simulink model "BLDC_Final"  (R2021b)
settings: Solver=odeN  StartTime=0.0  StopTime=5  MaxStep=Ts_motor  RelTol=1e-3  EnableMultiTasking=on
InitFcn:
  | load bldcData
model workspace (MAT data in the model file):
  encoderResolution = 2000
  hallOffset = '0.5'
  indexOffset = 850
  polePairs = '4'
undefined symbols (not defined in the file): DiscIntNeverNeededParam, Ts_motor, X, Y, Z
libraries: nesl_utility x23, ee_lib x8, fl_lib x8, sm_lib x7, spsPWMGeneratorDCDCLib x1, slpidlib x1, simulink_extras x1
(part 2 of 2)

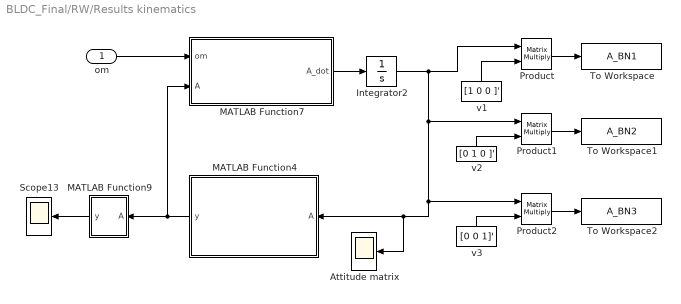
== system BLDC_Final/RW/Results kinematics ==
  om : Inport
  Attitude matrix : Scope
  Integrator2 : Integrator  InitialCondition=eye(3)
  MATLAB Function4 : MATLAB Function  TreatAsAtomicUnit=on
  MATLAB Function7 : MATLAB Function  TreatAsAtomicUnit=on
  MATLAB Function9 : MATLAB Function  TreatAsAtomicUnit=on
  Product : Product  Multiplication=Matrix(*)
  Product1 : Product  Multiplication=Matrix(*)
  Product2 : Product  Multiplication=Matrix(*)
  Scope13 : Scope
  To Workspace : ToWorkspace  VariableName=A_BN1  SampleTime=-1
  To Workspace1 : ToWorkspace  VariableName=A_BN2  SampleTime=-1
  To Workspace2 : ToWorkspace  VariableName=A_BN3  SampleTime=-1
  v1 : Constant  Value=[1 0 0 ]'
  v2 : Constant  Value=[0 1 0 ]'
  v3 : Constant  Value=[0 0 1]'
  wires:
  MATLAB Function7/1(A_dot) -> Integrator2/1
  MATLAB Function4/1(y) -> MATLAB Function9/1(A), MATLAB Function7/2(A)
  MATLAB Function9/1(y) -> Scope13/1
  om/1 -> MATLAB Function7/1(om)
  v1/1 -> Product/2
  Product/1 -> To Workspace/1
  Product1/1 -> To Workspace1/1
  v2/1 -> Product1/2
  v3/1 -> Product2/2
  Product2/1 -> To Workspace2/1
  Integrator2/1 -> Attitude matrix/1, MATLAB Function4/1(A), Product2/1, Product1/1, Product/1

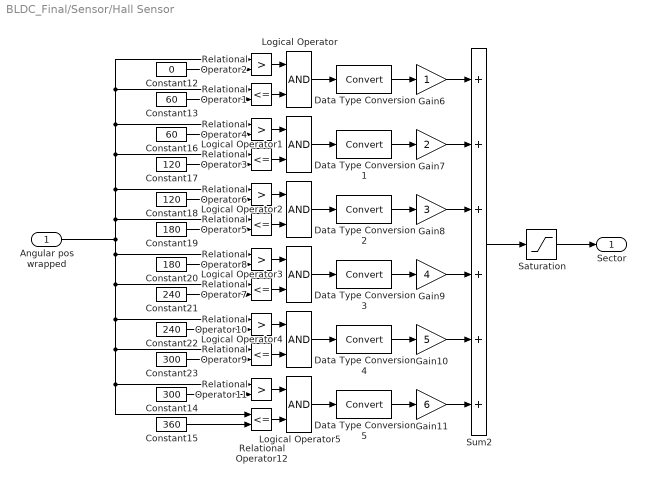
== system BLDC_Final/Sensor/Hall Sensor ==
  Angular pos wrapped : Inport
  Constant12 : Constant  Value=0
  Constant13 : Constant  Value=60
  Constant14 : Constant  Value=300
  Constant15 : Constant  Value=360
  Constant16 : Constant  Value=60
  Constant17 : Constant  Value=120
  Constant18 : Constant  Value=120
  Constant19 : Constant  Value=180
  Constant20 : Constant  Value=180
  Constant21 : Constant  Value=240
  Constant22 : Constant  Value=240
  Constant23 : Constant  Value=300
  Data Type Conversion{,1..5} (6 alike) : DataTypeConversion  SaturateOnIntegerOverflow=on  RndMeth=Zero
  Gain10 : Gain  Gain=5  SaturateOnIntegerOverflow=on  OutDataTypeStr=Inherit: Same as input  ParamDataTypeStr=Inherit: Same as input
  Gain11 : Gain  Gain=6  SaturateOnIntegerOverflow=on  OutDataTypeStr=Inherit: Same as input  ParamDataTypeStr=Inherit: Same as input
  Gain6 : Gain  SaturateOnIntegerOverflow=on  OutDataTypeStr=Inherit: Same as input  ParamDataTypeStr=Inherit: Same as input
  Gain7 : Gain  Gain=2  SaturateOnIntegerOverflow=on  OutDataTypeStr=Inherit: Same as input  ParamDataTypeStr=Inherit: Same as input
  Gain8 : Gain  Gain=3  SaturateOnIntegerOverflow=on  OutDataTypeStr=Inherit: Same as input  ParamDataTypeStr=Inherit: Same as input
  Gain9 : Gain  Gain=4  SaturateOnIntegerOverflow=on  OutDataTypeStr=Inherit: Same as input  ParamDataTypeStr=Inherit: Same as input
  Logical Operator{,1..5} (6 alike) : Logic
  Relational Operator{1,3,5,7,9,12} (6 alike) : RelationalOperator  Operator=<=  RndMeth=Nearest  InputSameDT=on
  Relational Operator{2,4,6,8,10..11} (6 alike) : RelationalOperator  Operator=>  RndMeth=Nearest  InputSameDT=on
  Saturation : Saturate  UpperLimit=6  LowerLimit=1
  Sum2 : Sum  Inputs=++++++  InputSameDT=on  SaturateOnIntegerOverflow=on  OutDataTypeStr=Inherit: Same as first input
  Sector : Outport
  wires:
  Relational Operator7/1 -> Logical Operator3/2
  Data Type Conversion/1 -> Gain6/1
  Relational Operator8/1 -> Logical Operator3/1
  Constant16/1 -> Relational Operator4/2
  Gain10/1 -> Sum2/5
  Gain7/1 -> Sum2/2
  Constant14/1 -> Relational Operator11/2
  Constant23/1 -> Relational Operator9/2
  Logical Operator1/1 -> Data Type Conversion1/1
  Constant22/1 -> Relational Operator10/2
  Constant20/1 -> Relational Operator8/2
  Relational Operator5/1 -> Logical Operator2/2
  Logical Operator2/1 -> Data Type Conversion2/1
  Data Type Conversion2/1 -> Gain8/1
  Constant12/1 -> Relational Operator2/2
  Gain6/1 -> Sum2/1
  Constant13/1 -> Relational Operator1/2
  Relational Operator12/1 -> Logical Operator5/2
  Relational Operator10/1 -> Logical Operator4/1
  Relational Operator6/1 -> Logical Operator2/1
  Data Type Conversion5/1 -> Gain11/1
  Relational Operator1/1 -> Logical Operator/2
  Data Type Conversion4/1 -> Gain10/1
  Gain8/1 -> Sum2/3
  Constant19/1 -> Relational Operator5/2
  Logical Operator3/1 -> Data Type Conversion3/1
  Constant21/1 -> Relational Operator7/2
  Logical Operator/1 -> Data Type Conversion/1
  Relational Operator4/1 -> Logical Operator1/1
  Constant17/1 -> Relational Operator3/2
  Relational Operator9/1 -> Logical Operator4/2
  Data Type Conversion1/1 -> Gain7/1
  Gain9/1 -> Sum2/4
  Relational Operator2/1 -> Logical Operator/1
  Relational Operator11/1 -> Logical Operator5/1
  Relational Operator3/1 -> Logical Operator1/2
  Logical Operator5/1 -> Data Type Conversion5/1
  Sum2/1 -> Saturation/1
  Constant15/1 -> Relational Operator12/2
  Data Type Conversion3/1 -> Gain9/1
  Constant18/1 -> Relational Operator6/2
  Gain11/1 -> Sum2/6
  Logical Operator4/1 -> Data Type Conversion4/1
  Saturation/1 -> Sector/1
  Angular pos wrapped/1 -> Relational Operator6/1, Relational Operator3/1, Relational Operator4/1, Relational Operator1/1, Relational Operator2/1, Relational Operator5/1, Relational Operator8/1, Relational Operator7/1, Relational Operator10/1, Relational Operator9/1, Relational Operator11/1, Relational Operator12/1

== system BLDC_Final/Sensor/wrapping ==
  Angular pos : Inport
  Constant3 : Constant  Value=360
  Gain1 : Gain  Gain=2
  Math Function : Math  Operator=rem  SignedPower=on  SaturateOnIntegerOverflow=on
  Unit Delay1 : UnitDelay  SampleTime=Ts_motor  HasFrameUpgradeWarning=on
  Angular pos wrapped : Outport
  tag scope: Angular_pos_wrapped=global
  wires:
  Constant3/1 -> Math Function/2
  Math Function/1 -> [Angular_pos_wrapped], Angular pos wrapped/1
  Angular pos/1 -> Gain1/1
  Gain1/1 -> Unit Delay1/1
  Unit Delay1/1 -> Math Function/1

== matlab function BLDC_Final/RW/Results kinematics/MATLAB Function7 ==
  data: om input; A_dot output; A input
function A_dot = Kinematics(om,A)
OM = [0 -om(3) om(2); om(3) 0 -om(1); -om(2) om(1) 0];

A_dot = -OM*A;

end

== matlab function BLDC_Final/RW/Results kinematics/MATLAB Function4 ==
  data: A input; y output
function y= orthoex(A)
for k =1:3
A_ex = A * 3/2 - A * A'* A/2;  % a way to correct the error of no orthonormalization
end
y = A_ex;
end

== matlab function BLDC_Final/RW/Results kinematics/MATLAB Function9 ==
  data: A input; y output
function y = control(A)
y = det(A);

end
